simulink model "t1q3"  (R2017b)
settings: Solver=VariableStepAuto  StartTime=0.0  StopTime=10.0  RelTol=1e-3
values from neighbouring files (symbols this model uses):
  Ca_0 = 0.7192    [t1.m]    (also in t1q5.m = double(max(solve(0 == -k1*Ca - k3*Ca^2 + (Caf_0 - Ca)*u_0,Ca; t1q9.m = double(max(solve(0 == -k1*Ca - k3*Ca^2 + (Caf_0 - Ca)*u_0,Ca)
  Caf_0 = 5.1    [t1.m]    (also in t1q5.m; t1q9.m)
  Cb_0 = 2.345    [t1.m]    (also in t1q5.m = double(solve(0 == k1*Ca_0 - k2*Cb - Cb*u_0, Cb)); t1q9.m = double(solve(0 == k1*Ca_0 - k2*Cb - Cb*u_0, Cb)))
  k1 = 6.01    [t1.m]    (also in t1q5.m; t1q9.m)
  k2 = 0.8433    [t1.m]    (also in t1q5.m; t1q9.m)
  k3 = 0.1123    [t1.m]    (also in t1q5.m; t1q9.m)
  u_0 = 1    [t1.m]    (also in t1q5.m; t1q9.m)
libraries: cstblocks x4
settings Model: Creator=vinic  LastModifiedBy=vinic

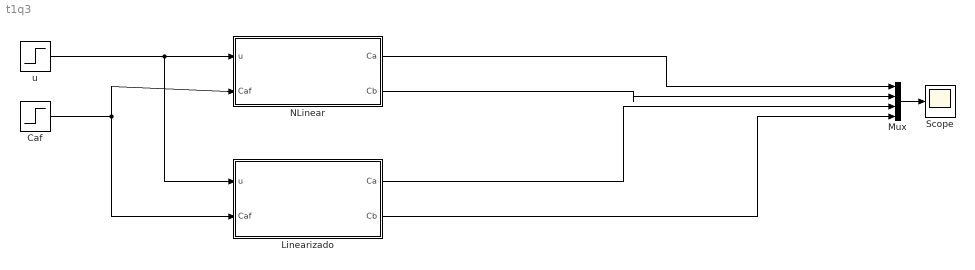
== system t1q3 ==
  Caf : Step  Time=5  Before=5.1  After=5.2  SampleTime=0
  Linearizado : Subsystem
  Mux : Mux
  NLinear : Subsystem
  Scope : Scope
  u : Step  Before=1  After=1.1  SampleTime=0
  wires:
  Mux/1 -> Scope/1
  u/1 -> Linearizado/1(u), NLinear/1(u)
  Caf/1 -> NLinear/2(Caf), Linearizado/2(Caf)
  NLinear/1(Ca) -> Mux/1
  NLinear/2(Cb) -> Mux/2
  Linearizado/1(Ca) -> Mux/3
  Linearizado/2(Cb) -> Mux/4

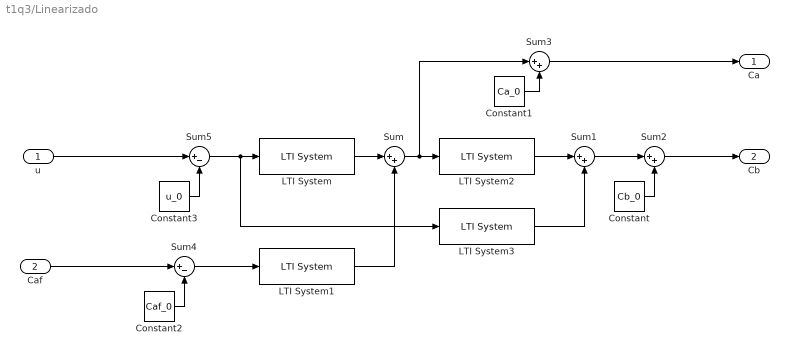
== system t1q3/Linearizado ==
  u : Inport
  Caf : Inport  Port=2
  Constant : Constant  Value=Cb_0
  Constant1 : Constant  Value=Ca_0
  Constant2 : Constant  Value=Caf_0
  Constant3 : Constant  Value=u_0
  LTI System : cstblocks/LTI System  sys=Ca_U  IC=[]
  LTI System1 : cstblocks/LTI System  sys=Ca_Caf  IC=[]
  LTI System2 : cstblocks/LTI System  sys=Cb_Ca  IC=[]
  LTI System3 : cstblocks/LTI System  sys=Cb_U  IC=[]
  Sum{,1..3} (4 alike) : Sum  Inputs=|++
  Sum4 : Sum  Inputs=|+-
  Sum5 : Sum  Inputs=|+-
  Ca : Outport
  Cb : Outport  Port=2
  wires:
  Sum1/1 -> Sum2/1
  Sum5/1 -> LTI System3/1, LTI System/1
  Sum4/1 -> LTI System1/1
  Constant2/1 -> Sum4/2
  Constant3/1 -> Sum5/2
  LTI System1/1 -> Sum/2
  LTI System/1 -> Sum/1
  Sum3/1 -> Ca/1
  Sum2/1 -> Cb/1
  LTI System2/1 -> Sum1/1
  Constant1/1 -> Sum3/2
  LTI System3/1 -> Sum1/2
  Constant/1 -> Sum2/2
  Sum/1 -> Sum3/1, LTI System2/1
  u/1 -> Sum5/1
  Caf/1 -> Sum4/1

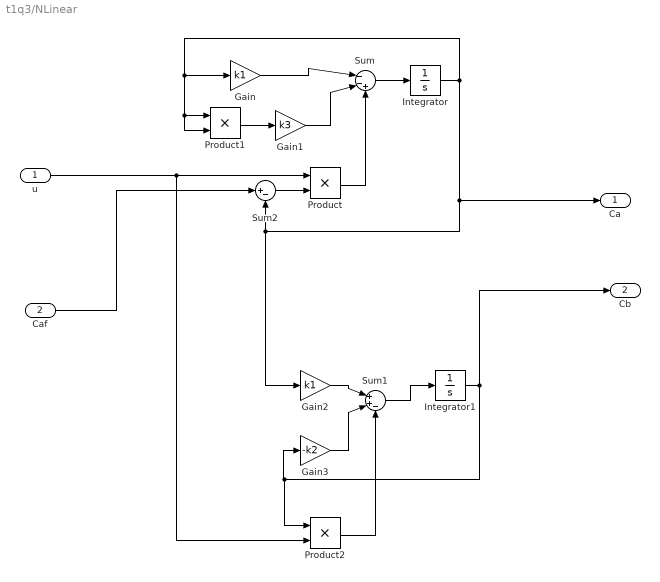
== system t1q3/NLinear ==
  u : Inport
  Caf : Inport  Port=2
  Gain : Gain  Gain=k1
  Gain1 : Gain  Gain=k3
  Gain2 : Gain  Gain=k1
  Gain3 : Gain  Gain=-k2
  Integrator : Integrator  InitialCondition=Ca_0
  Integrator1 : Integrator  InitialCondition=Cb_0
  Product : Product
  Product1 : Product
  Product2 : Product
  Sum : Sum  Inputs=|--+
  Sum1 : Sum  Inputs=|++-
  Sum2 : Sum  Inputs=|+-
  Ca : Outport
  Cb : Outport  Port=2
  wires:
  Sum/1 -> Integrator/1
  Integrator1/1 -> Cb/1, Product2/1, Gain3/1
  Caf/1 -> Sum2/1
  u/1 -> Product2/2, Product/1
  Integrator/1 -> Ca/1, Gain2/1, Sum2/2, Product1/1, Product1/2, Gain/1
  Sum2/1 -> Product/2
  Gain/1 -> Sum/1
  Product/1 -> Sum/3
  Gain3/1 -> Sum1/2
  Product2/1 -> Sum1/3
  Sum1/1 -> Integrator1/1
  Gain1/1 -> Sum/2
  Product1/1 -> Gain1/1
  Gain2/1 -> Sum1/1
